simulink model "qc_quarter_car_lqr_discrete"  (R2024b)
settings: Solver=FixedStepDiscrete  StartTime=0.0  StopTime=20  FixedStep=dt  RelTol=1e-3
model workspace (MAT data in the model file):
  Ad_a = [0.999994576097  2.73384593354e-05  0.000371068048286  4.30917358955e-07; -0.00274343856749  0.00221477741281  0.186704480516  0.000403340055634; 3.00631230622e-05  0.0109338910714  0.990840599431  0.00199287182416; 0.0151355945438  5.5047972031  -8.12427099654  0.990662554249]
  Ad_p = [0.999874224795  0.0019920548301  0.000106923063305  7.93573182678e-06; -0.124669915588  0.99208235507  0.096453980204  0.00789879278756; 0.000697917546571  4.40873990377e-05  0.992304054846  0.00195122763912; 0.690948233705  0.0438821821531  -7.62864650613  0.949119790239]
  Bd_a = [1.08435901706e-06; 0.00153215060962; 0.00709666766388; 7.0857664859]
  Bd_p = [7.86095033855e-09  1.88521421122e-05; 7.79186972425e-06  0.0282159353841; -4.36198466607e-08  0.00699802760782; -4.31842646065e-05  6.93769827243]
  K_lqr = [11495.4541697 9999008.40234 -1870556.42794 676.5615569]
  Q = [500  0  0  0; 0  100000000  0  0; 0  0  100  0; 0  0  0  1000]
  R = 1e-06
  b1 = 1000
  b2 = 0
  dt = 0.002
  k1 = 16000
  k2 = 160000
  m1 = 250
  m2 = 45
settings Model: Creator=abdel  LastModifiedBy=abdel

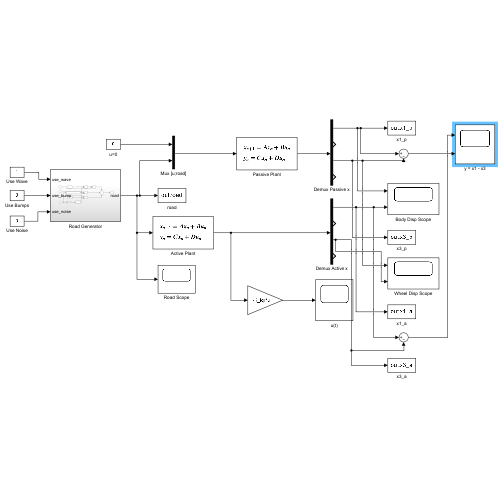
[thumbnail: Simulink's stored preview of the top-level diagram]
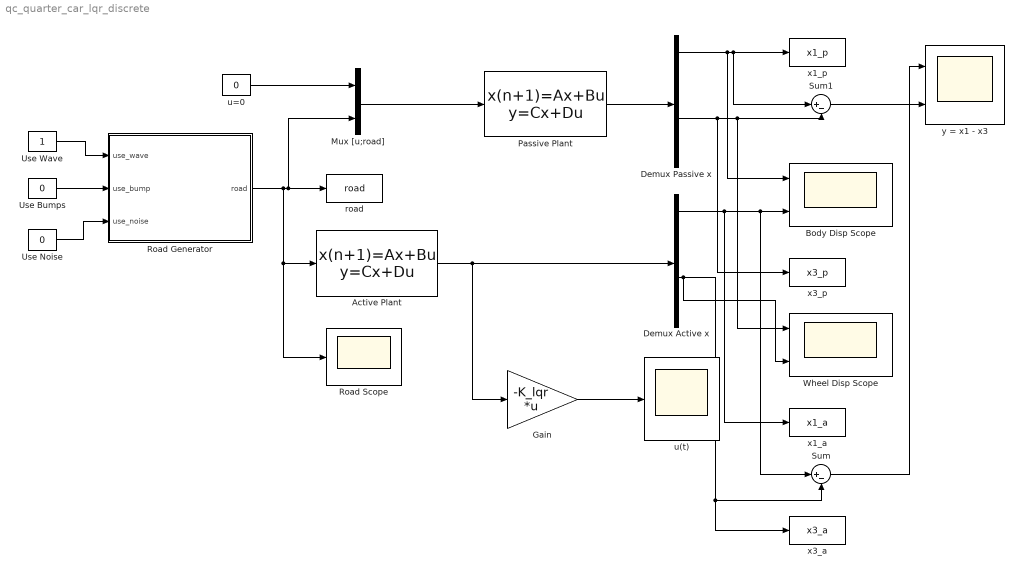
== system qc_quarter_car_lqr_discrete ==
  Active Plant : DiscreteStateSpace  A=Ad_a  B=Bd_a  C=eye(4)  D=zeros(4,1)  InitialCondition=zeros(4,1)  SampleTime=dt
  Body Disp Scope : Scope  NumInputPorts=2
  Demux Active x : Demux
  Demux Passive x : Demux
  Gain : Gain  Gain=-K_lqr  Multiplication=Matrix(K*u)
  Mux [u;road] : Mux  Inputs=2
  Passive Plant : DiscreteStateSpace  A=Ad_p  B=Bd_p  C=eye(4)  D=zeros(4,2)  InitialCondition=zeros(4,1)  SampleTime=dt
  Road Generator : Subsystem
  Road Scope : Scope
  Sum : Sum  Inputs=|+-
  Sum1 : Sum  Inputs=|+-
  Use Bumps : Constant  Value=0
  Use Noise : Constant  Value=0
  Use Wave : Constant
  Wheel Disp Scope : Scope  NumInputPorts=2
  road : ToWorkspace  VariableName=road  SaveFormat=Timeseries  SampleTime=-1
  u(t) : Scope
  u=0 : Constant  Value=0
  x1_a : ToWorkspace  VariableName=x1_a  SaveFormat=Timeseries  SampleTime=-1
  x1_p : ToWorkspace  VariableName=x1_p  SaveFormat=Timeseries  SampleTime=-1
  x3_a : ToWorkspace  VariableName=x3_a  SaveFormat=Timeseries  SampleTime=-1
  x3_p : ToWorkspace  VariableName=x3_p  SaveFormat=Timeseries  SampleTime=-1
  y = x1 - x3 : Scope  NumInputPorts=2
  wires:
  Passive Plant/1 -> Demux Passive x/1
  Use Wave/1 -> Road Generator/1(use_wave)
  Use Bumps/1 -> Road Generator/2(use_bump)
  Active Plant/1 -> Demux Active x/1, Gain/1
  Sum/1 -> y = x1 - x3/1
  Sum1/1 -> y = x1 - x3/2
  Use Noise/1 -> Road Generator/3(use_noise)
  Mux [u;road]/1 -> Passive Plant/1
  u=0/1 -> Mux [u;road]/1
  Road Generator/1(road) -> Active Plant/1, Road Scope/1, road/1, Mux [u;road]/2
  Gain/1 -> u(t)/1
  Demux Passive x/1 -> x1_p/1, Sum1/1, Body Disp Scope/1
  Demux Passive x/3 -> Sum1/2, Wheel Disp Scope/1, x3_p/1
  Demux Active x/1 -> Body Disp Scope/2, Sum/1, x1_a/1
  Demux Active x/3 -> Sum/2, x3_a/1, Wheel Disp Scope/2

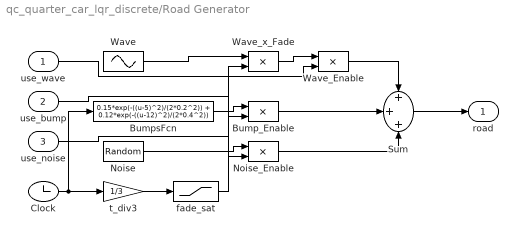
== system qc_quarter_car_lqr_discrete/Road Generator ==
  use_wave : Inport
  use_bump : Inport  Port=2
  use_noise : Inport  Port=3
  Bump_Enable : Product
  BumpsFcn : Fcn  Expr=0.15*exp(-((u-5)^2)/(2*0.2^2)) + 0.12*exp(-((u-12)^2)/(2*0.4^2))
  Clock : Clock
  Noise : RandomNumber  Variance=0.015^2  Seed=1  SampleTime=dt
  Noise_Enable : Product
  Sum : Sum  Inputs=+++
  Wave : Sin  Amplitude=0.1  Frequency=2*pi*1.27  SampleTime=dt
  Wave_Enable : Product
  Wave_x_Fade : Product
  fade_sat : Saturate  UpperLimit=1  LowerLimit=0
  t_div3 : Gain  Gain=1/3
  road : Outport
  wires:
  Clock/1 -> t_div3/1, BumpsFcn/1
  t_div3/1 -> fade_sat/1
  Wave/1 -> Wave_x_Fade/1
  fade_sat/1 -> Wave_x_Fade/2
  Wave_x_Fade/1 -> Wave_Enable/1
  use_wave/1 -> Wave_Enable/2
  BumpsFcn/1 -> Bump_Enable/1
  use_bump/1 -> Bump_Enable/2
  Noise/1 -> Noise_Enable/1
  use_noise/1 -> Noise_Enable/2
  Wave_Enable/1 -> Sum/1
  Bump_Enable/1 -> Sum/2
  Noise_Enable/1 -> Sum/3
  Sum/1 -> road/1
